simulink model "ReachTask_Perturb"  (R2022b)
settings: Solver=FixedStepDiscrete  StartTime=0.0  StopTime=Inf  FixedStep=0.001  RelTol=1e-3  EnableMultiTasking=on
PreLoadFcn:
  | parambus = Simulink.Bus;
  | idx = 0;
  | 
  | idx = idx + 1;
  | parambus.Elements(idx) = Simulink.BusElement;
  | parambus.Elements(idx).Name = 'ScreenOn';
  | parambus.Elements(idx).DataType = 'uint8';
  | parambus.Elements(idx).Dimensions = [1, 1];
  | 
  | idx = idx + 1;
  | parambus.Elements(idx) = Simulink.BusElement;
  | parambus.Elements(idx).Name = 'DelayPeriod';
  | parambus.Elements(idx).DataType = 'uint16';
  | parambus.Elements(idx).Dimensions = [1, 2];
  | 
  | idx = idx + 1;
  | parambus.Elements(idx) = Simulink.BusElement;
  | parambus.Elements(idx).Name = 'TargetHoldTime';
  | parambus.Elements(idx).DataType = 'uint16';
  | parambus.Elements(idx).Dimensions = [1, 1];
  | 
  | idx = idx + 1;
  | parambus.Elements(idx) = Simulink.BusElement;
  | parambus.Elements(idx).Name = 'TargetScaling';
  | parambus.Elements(idx).DataType = 'uint8';
  | parambus.Elements(idx).Dimensions = [1, 1];
  | 
  | idx = idx + 1;
  | parambus.Elements(idx) = Simulink.BusElement;
  | parambus.Elements(idx).Name = 'TrialTimeout';
  | parambus.Elements(idx).DataType = 'uint16';
  | parambus.Elements(idx).Dimensions = [1, 1];
  | 
  | 
  | FileLoggerEntry = Simulink.Bus;
  | FileLoggerEntry.Elements(1) = Simulink.BusElement;
  | FileLoggerEntry.Elements(1).Name = 'FileType';
  | FileLoggerEntry.Elements(1).DataType = 'uint8';
  | FileLoggerEntry.Elements(1).Dimensions = [1, 1];
  | FileLoggerEntry.Elements(2) = Simulink.BusElement;
  | FileLoggerEntry.Elements(2).Name = 'FieldName';
  | FileLoggerEntry.Elements(2).DataType = 'uint8';
  | FileLoggerEntry.Elements(2).Dimensions = [1, 20];
  | FileLoggerEntry.Elements(3) = Simulink.BusElement;
  | FileLoggerEntry.Elements(3).Name = 'DataType';
  | FileLoggerEntry.Elements(3).DataType = 'uint8';
  | FileLoggerEntry.Elements(3).Dimensions = [1, 6];
  | FileLoggerEntry.Elements(4) = Simulink.BusElement;
  | FileLoggerEntry.Elements(4).Name = 'NumElements';
  | FileLoggerEntry.Elements(4).DataType = 'uint8';
  | FileLoggerEntry.Elements(4).Dimensions = [1, 1];
  | FileLoggerEntry.Elements(5) = Simulink.BusElement;
  | FileLoggerEntry.Elements(5).Name = 'Data';
  | FileLoggerEntry.Elements(5).DataType = 'double';
  | FileLoggerEntry.Elements(5).Dimensions = [1, 255];
undefined symbols (not defined in the file): IO397
libraries: slrealtimeiplib x7, speedgoatlib_fpga_spi x1, speedgoatlib_fpga x1
settings Model: Creator=irwin  LastModifiedBy=irwin
settings SolverCC: ConcurrentTasks=on  AlgebraicLoopSolver=TrustRegion  PositivePriorityOrder=on  InsertRTBMode=Never (minimum delay)
settings DataIOCC: SaveFormat=Array  SaveState=on  SignalLoggingName=logsOut
settings OptimizationCC: BlockReduction=off  BooleanDataType=off  OptimizeBlockIOStorage=off  BufferReuse=off  GlobalBufferReuse=off  ExpressionFolding=off  LocalBlockOutputs=off  InitFltsAndDblsToZero=on  OptimizeDataStoreBuffers=off  BusAssignmentInplaceUpdate=off
settings DebuggingCC: SaveWithParameterizedLinksMsg=none  UnderspecifiedInitializationDetection=Classic  MergeDetectMultiDrivingBlocksExec=none  CheckExecutionContextPreStartOutputMsg=on  SignalResolutionControl=TryResolveAllWithWarning  TasksWithSamePriorityMsg=none  UnconnectedInputMsg=warning  UnconnectedOutputMsg=warning  UnconnectedLineMsg=warning  SFUnexpectedBacktrackingDiag=warning  SFNoUnconditionalDefaultTransitionDiag=warning  SFExecutionAtInitializationDiag=none  SFMachineParentedDataDiag=warning  ArithmeticOperatorsInVariantConditions=warning
settings HardwareCC: ProdBitPerLong=64  ProdLongLongMode=on  ProdHWDeviceType=Intel->x86-64 (Linux 64)
settings ModelReferenceCC: EnableRefExpFcnMdlSchedulingChecks=on  PropagateSignalLabelsOutOfModel=off
settings SFSimCC: SimUseLocalCustomCode=off  SimTargetLang=C++
settings RTWCC: Description=Simulink Real-Time  SystemTargetFile=slrealtime.tlc  TemplateMakefile=slrealtime_default_tmf  RTWUseLocalCustomCode=off  Toolchain=Simulink Real-Time Toolchain  BuildConfiguration=Faster Runs  CodeExecutionProfiling=on  TargetLang=C++  DLArmComputeVersion=19.05
settings CodeAppCC: StateflowObjectComments=on
settings SimulinkRealTimeTargetCC: MATLABClassNameForMDSCustomization=Simulink.SoftwareTarget.GRTCustomization  UseGCCFastMath=on
settings ConfigComp: CovMetricSettings=dw  CovSaveCumulativeToWorkspaceVar=on  CovSaveSingleToWorkspaceVar=on  CovExternalEMLEnable=off  CovSFcnEnable=off

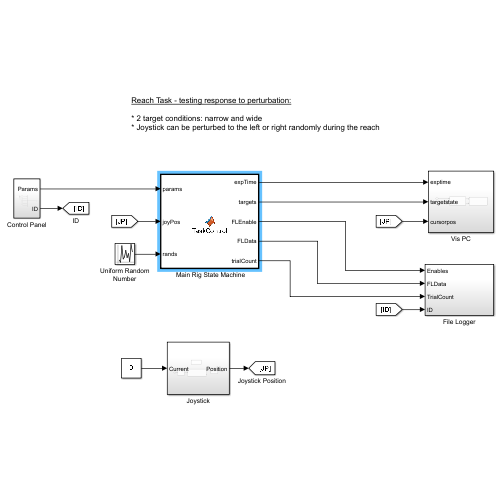
[thumbnail: Simulink's stored preview of the top-level diagram]
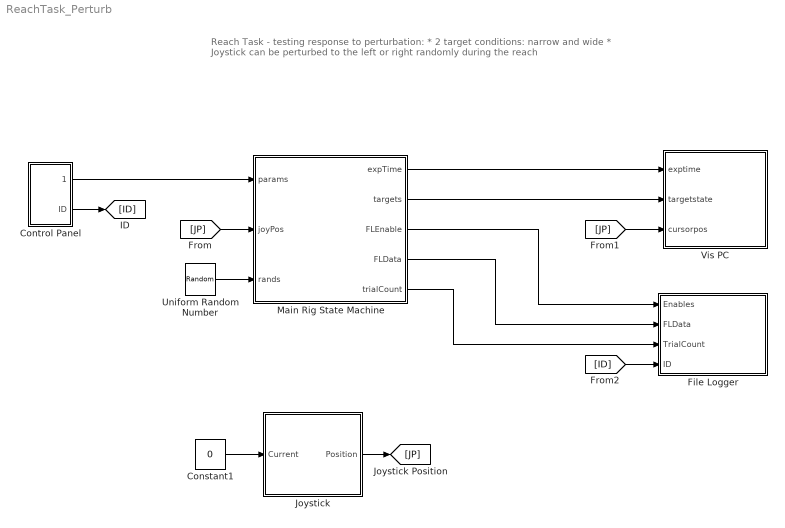
== system ReachTask_Perturb ==
  note: Reach Task - testing response to perturbation:
      |
      | * 2 target conditions: narrow and wide
      | * Joystick can be perturbed to the left or right randomly during the reach
  " Main Rig State Machine" : MATLAB Function  TreatAsAtomicUnit=on
  Constant1 : Constant  Value=0  OutMin=-5  OutMax=5  OutDataTypeStr=single
  Control Panel : Subsystem
  File Logger : Subsystem
  Joystick : Subsystem
  Uniform Random Number : UniformRandomNumber  Minimum=[0, 0, 0]  Maximum=[2, 2, 1]  SampleTime=.001
  Vis PC : Subsystem
  wires:
  " Main Rig State Machine"/1(expTime) -> Vis PC/1(exptime)
  " Main Rig State Machine"/2(targets) -> Vis PC/2(targetstate)
  " Main Rig State Machine"/3(FLEnable) -> File Logger/1(Enables)
  " Main Rig State Machine"/4(FLData) -> File Logger/2(FLData)
  " Main Rig State Machine"/5(trialCount) -> File Logger/3(TrialCount)
  [JP] -> " Main Rig State Machine"/2(joyPos)
  [JP] -> Vis PC/3(cursorpos)
  Control Panel/2(ID) -> [ID]
  [ID] -> File Logger/4(ID)
  Control Panel/1(Params) -> " Main Rig State Machine"/1(params)
  Uniform Random Number/1 -> " Main Rig State Machine"/3(rands)
  Joystick/1(Position) -> [JP]
  Constant1/1 -> Joystick/1(Current)

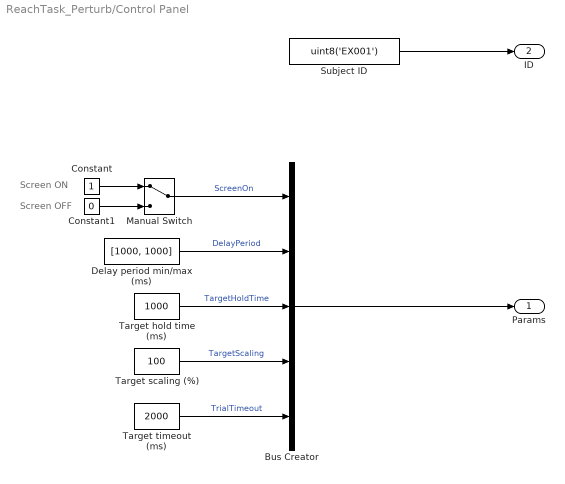
== system ReachTask_Perturb/Control Panel ==
  note: Screen ON
  note: Screen OFF
  Bus Creator : BusCreator  Inputs=5  OutDataTypeStr=Bus: parambus  NonVirtualBus=on
      settings: InheritFromInputs=off
  Constant : Constant  OutDataTypeStr=uint8
  Constant1 : Constant  Value=0  OutDataTypeStr=uint8
  Delay period min/max (ms) : Constant  Value=[1000, 1000]  OutDataTypeStr=uint16
  Manual Switch : ManualSwitch
  Subject ID : Constant  Value=uint8('EX001')  OutDataTypeStr=uint8
  Target hold time (ms) : Constant  Value=1000  OutDataTypeStr=uint16
  Target scaling (%) : Constant  Value=100  OutDataTypeStr=uint8
  Target timeout (ms) : Constant  Value=2000  OutDataTypeStr=uint16
  Params : Outport
  ID : Outport  Port=2
  wires:
  Delay period min/max (ms)/1 -> Bus Creator/2  "DelayPeriod"
  Manual Switch/1 -> Bus Creator/1  "ScreenOn"
  Constant1/1 -> Manual Switch/2
  Constant/1 -> Manual Switch/1
  Bus Creator/1 -> Params/1
  Target hold time (ms)/1 -> Bus Creator/3  "TargetHoldTime"
  Subject ID/1 -> ID/1
  Target timeout (ms)/1 -> Bus Creator/5  "TrialTimeout"
  Target scaling (%)/1 -> Bus Creator/4  "TargetScaling"

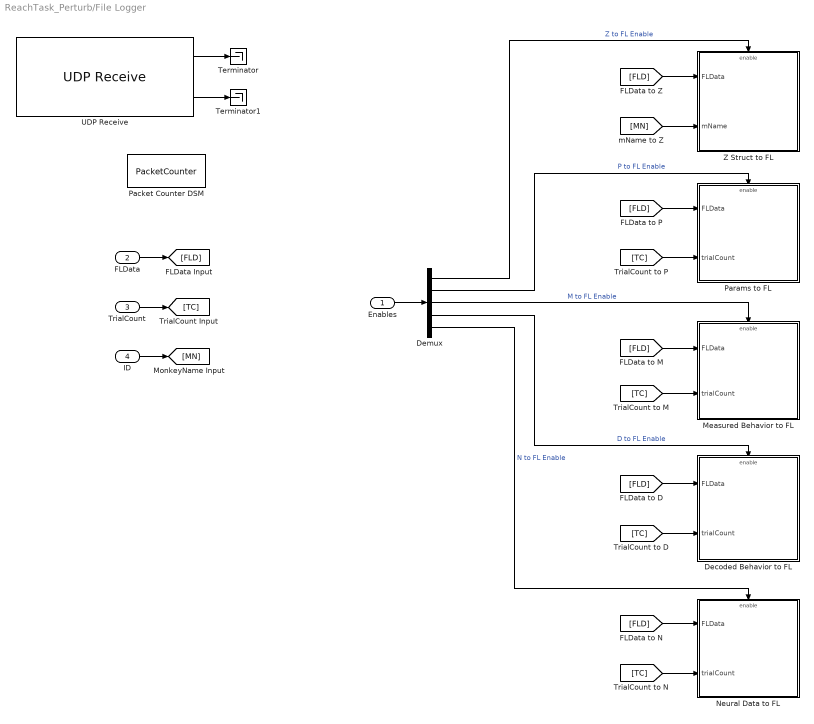
== system ReachTask_Perturb/File Logger ==
  Enables : Inport  OutDataTypeStr=uint8  PortDimensions=[1 5]
  FLData : Inport  Port=2  OutDataTypeStr=Bus: FileLoggerEntry
  TrialCount : Inport  Port=3
  ID : Inport  Port=4
  Decoded Behavior to FL : Subsystem
  Demux : Demux  Outputs=5
  Measured Behavior to FL : Subsystem
  Neural Data to FL : Subsystem
  Packet Counter DSM : DataStoreMemory  DataStoreName=PacketCounter  WriteAfterWriteMsg=warning  ShowAdditionalParam=off  OutDataTypeStr=uint32  Dimensions=1
  Params to FL : Subsystem
  Terminator : Terminator
  Terminator1 : Terminator
  UDP Receive : slrealtimeiplib/UDP Receive  useHostTargetConn=off  ipAddress='192.168.8.1'  localPort=11114  rcvWidth=16  rcvFmAny=off  fmAddress='192.168.8.7'  sampleTime=-1  enableMessage=off  maxPackets=1
  Z Struct to FL : Subsystem
  wires:
  TrialCount/1 -> [TC]
  FLData/1 -> [FLD]
  [FLD] -> Z Struct to FL/1(FLData)
  [FLD] -> Params to FL/1(FLData)
  [FLD] -> Measured Behavior to FL/1(FLData)
  [FLD] -> Decoded Behavior to FL/1(FLData)
  [FLD] -> Neural Data to FL/1(FLData)
  [TC] -> Params to FL/2(trialCount)
  [TC] -> Measured Behavior to FL/2(trialCount)
  [TC] -> Decoded Behavior to FL/2(trialCount)
  [TC] -> Neural Data to FL/2(trialCount)
  Enables/1 -> Demux/1
  Demux/3 -> Measured Behavior to FL/Enable  "M to FL Enable"
  Demux/4 -> Decoded Behavior to FL/Enable  "D to FL Enable"
  Demux/5 -> Neural Data to FL/Enable  "N to FL Enable"
  Demux/2 -> Params to FL/Enable  "P to FL Enable"
  Demux/1 -> Z Struct to FL/Enable  "Z to FL Enable"
  ID/1 -> [MN]
  [MN] -> Z Struct to FL/2(mName)
  UDP Receive/2 -> Terminator1/1
  UDP Receive/1 -> Terminator/1

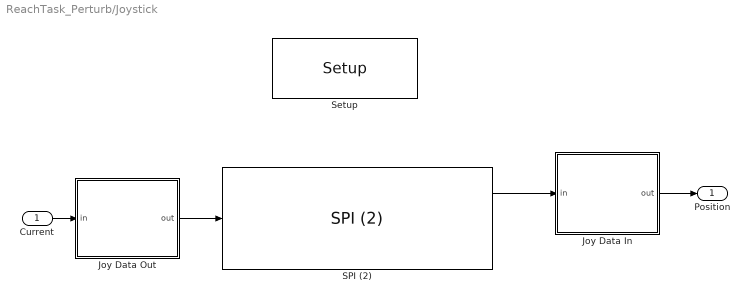
== system ReachTask_Perturb/Joystick ==
  Current : Inport
  Joy Data In : MATLAB Function  TreatAsAtomicUnit=on
  Joy Data Out : MATLAB Function  TreatAsAtomicUnit=on
  SPI (2) : speedgoatlib_fpga_spi/SPI (2)  id=1  chan=[1]  samp_time=.001  board=IO397-50k  pciSlot=-1  role=Master  sync_mode=off  multislave_mode=off  write_only=off  read_only=off  multislave_chan=[1]  cpol=[0]  cpha=[0]  frequency=[1e6]  frequency_eff=1e6  delay_start=[2e-6]  delay_start_eff=2e-6  delay_interword=[1e-6]  delay_interword_eff=1e-6  delay_stop=[1e-6]  delay_stop_eff=1e-6  delay_compensation=[100e-9]  delay_compensation_eff=106.7e-9  words_per_frame=[2]  dynamic_words_per_frame=off  bits_per_word=[16]  bit_shift_lsb_first=[0]  no_cs=off  clock_timeout=[1e-6]  clock_timeout_eff=1E-06
      settings: SourceProductName=Simulink Real-Time: Speedgoat I/O Blockset
  Setup : speedgoatlib_fpga/Setup/Setup  board=IO397-50k  id=1  device_id=1  frontIO=None  rearIO=None  bitstreamFile=speedgoat_IO397_50k_Comms.mat  rev=4.000000  timestamp_string=18/02/22 13:58:38  fpgaFreq=75 MHz  fpgaTick=13.33 ns  ProgSpiFlash=off  ProgBPIFlash=off  pciSlot=-1  PullRPort0=pull-up 3.3V  VioPort0=3.3V  PullRPort1=pull-up 3.3V  VioPort1=3.3V  PullRPort2=pull-up 3.3V  VioPort2=3.3V  PullRPort3=pull-up 3.3V  VioPort3=3.3V  PullRPort4=pull-up 3.3V  VioPort4=3.3V  PullRPort5=pull-up 3.3V  VioPort5=3.3V  PullRPort6=pull-up 3.3V  VioPort6=3.3V  diffLineTermination_rear1=on  diffLineTermination_rear2=on  diffLineTermination_rear3=on  diffLineTermination_rear4=on  diffLineTermination_rear5=on  diffLineTermination_rear6=on  diffLineTermination_rear7=on  diffLineTermination_rear8=on  PullRPort15=pull-up 3.3V  PullRPort31=pull-up 3.3V  PullRPort47=pull-up 3.3V  PullRPort63=pull-up 3.3V  diffLineTermination_1=on  diffLineTermination_2=on  diffLineTermination_3=on  diffLineTermination_4=on  diffLineTermination_5=on  diffLineTermination_6=on  diffLineTermination_7=on  diffLineTermination_8=on
      settings: SourceProductName=Simulink Real-Time: Speedgoat I/O Blockset
  Position : Outport
  wires:
  Joy Data Out/1(out) -> SPI (2)/1
  SPI (2)/1 -> Joy Data In/1(in)
  Current/1 -> Joy Data Out/1(in)
  Joy Data In/1(out) -> Position/1

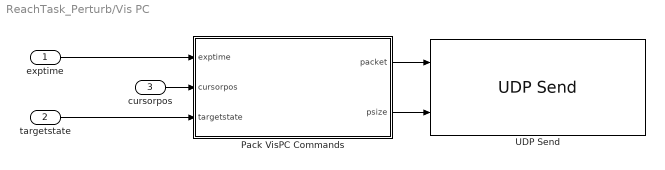
== system ReachTask_Perturb/Vis PC ==
  exptime : Inport
  targetstate : Inport  Port=2
  cursorpos : Inport  Port=3
  Pack VisPC Commands : MATLAB Function  TreatAsAtomicUnit=on
  UDP Send : slrealtimeiplib/UDP Send  useHostTargetConn=off  toAddress='192.168.11.6'  toPort=11114  sampleTime=-1  enableMessage=off  ipAddress='192.168.11.1'  localPort=11114
  wires:
  cursorpos/1 -> Pack VisPC Commands/2(cursorpos)
  Pack VisPC Commands/1(packet) -> UDP Send/1
  Pack VisPC Commands/2(psize) -> UDP Send/2
  targetstate/1 -> Pack VisPC Commands/3(targetstate)
  exptime/1 -> Pack VisPC Commands/1(exptime)

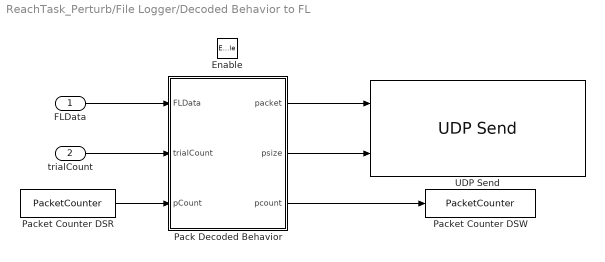
== system ReachTask_Perturb/File Logger/Decoded Behavior to FL ==
  FLData : Inport
  trialCount : Inport  Port=2
  Enable : EnablePort
  Pack Decoded Behavior : MATLAB Function  TreatAsAtomicUnit=on
  Packet Counter DSR : DataStoreRead  DataStoreName=PacketCounter  SampleTime=.001  IndexOptions=Index vector (dialog)  Indices=1  OutputSizes=1
  Packet Counter DSW : DataStoreWrite  DataStoreName=PacketCounter  IndexOptions=Index vector (dialog)  Indices=1  OutputSizes=1
  UDP Send : slrealtimeiplib/UDP Send  useHostTargetConn=off  toAddress='192.168.8.7'  toPort=11114  sampleTime=-1  enableMessage=off  ipAddress='192.168.8.1'  localPort=11114
  wires:
  FLData/1 -> Pack Decoded Behavior/1(FLData)
  trialCount/1 -> Pack Decoded Behavior/2(trialCount)
  Packet Counter DSR/1 -> Pack Decoded Behavior/3(pCount)
  Pack Decoded Behavior/1(packet) -> UDP Send/1
  Pack Decoded Behavior/3(pcount) -> Packet Counter DSW/1
  Pack Decoded Behavior/2(psize) -> UDP Send/2

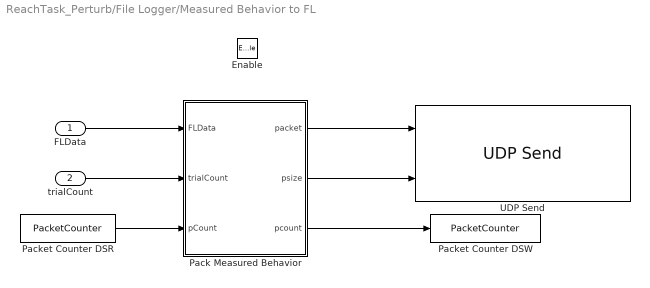
== system ReachTask_Perturb/File Logger/Measured Behavior to FL ==
  FLData : Inport
  trialCount : Inport  Port=2
  Enable : EnablePort
  Pack Measured Behavior : MATLAB Function  TreatAsAtomicUnit=on
  Packet Counter DSR : DataStoreRead  DataStoreName=PacketCounter  SampleTime=.001  IndexOptions=Index vector (dialog)  Indices=1  OutputSizes=1
  Packet Counter DSW : DataStoreWrite  DataStoreName=PacketCounter  IndexOptions=Index vector (dialog)  Indices=1  OutputSizes=1
  UDP Send : slrealtimeiplib/UDP Send  useHostTargetConn=off  toAddress='192.168.8.7'  toPort=11114  sampleTime=-1  enableMessage=off  ipAddress='192.168.8.1'  localPort=11114
  wires:
  FLData/1 -> Pack Measured Behavior/1(FLData)
  trialCount/1 -> Pack Measured Behavior/2(trialCount)
  Packet Counter DSR/1 -> Pack Measured Behavior/3(pCount)
  Pack Measured Behavior/3(pcount) -> Packet Counter DSW/1
  Pack Measured Behavior/1(packet) -> UDP Send/1
  Pack Measured Behavior/2(psize) -> UDP Send/2

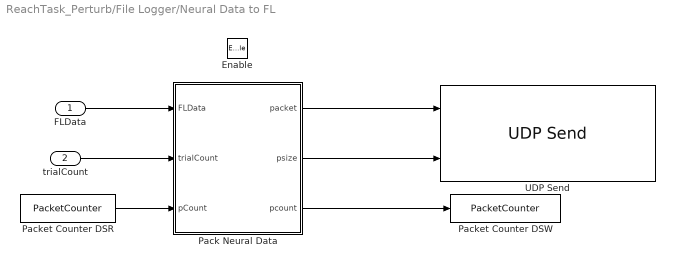
== system ReachTask_Perturb/File Logger/Neural Data to FL ==
  FLData : Inport
  trialCount : Inport  Port=2
  Enable : EnablePort
  Pack Neural Data : MATLAB Function  TreatAsAtomicUnit=on
  Packet Counter DSR : DataStoreRead  DataStoreName=PacketCounter  SampleTime=.001  IndexOptions=Index vector (dialog)  Indices=1  OutputSizes=1
  Packet Counter DSW : DataStoreWrite  DataStoreName=PacketCounter  IndexOptions=Index vector (dialog)  Indices=1  OutputSizes=1
  UDP Send : slrealtimeiplib/UDP Send  useHostTargetConn=off  toAddress='192.168.8.7'  toPort=11114  sampleTime=-1  enableMessage=off  ipAddress='192.168.8.1'  localPort=11114
  wires:
  FLData/1 -> Pack Neural Data/1(FLData)
  trialCount/1 -> Pack Neural Data/2(trialCount)
  Packet Counter DSR/1 -> Pack Neural Data/3(pCount)
  Pack Neural Data/3(pcount) -> Packet Counter DSW/1
  Pack Neural Data/1(packet) -> UDP Send/1
  Pack Neural Data/2(psize) -> UDP Send/2

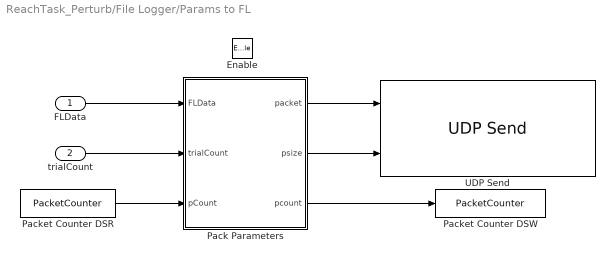
== system ReachTask_Perturb/File Logger/Params to FL ==
  FLData : Inport
  trialCount : Inport  Port=2
  Enable : EnablePort
  Pack Parameters : MATLAB Function  TreatAsAtomicUnit=on
  Packet Counter DSR : DataStoreRead  DataStoreName=PacketCounter  SampleTime=.001  IndexOptions=Index vector (dialog)  Indices=1  OutputSizes=1
  Packet Counter DSW : DataStoreWrite  DataStoreName=PacketCounter  IndexOptions=Index vector (dialog)  Indices=1  OutputSizes=1
  UDP Send : slrealtimeiplib/UDP Send  useHostTargetConn=off  toAddress='192.168.8.7'  toPort=11114  sampleTime=-1  enableMessage=off  ipAddress='192.168.8.1'  localPort=11114
  wires:
  FLData/1 -> Pack Parameters/1(FLData)
  trialCount/1 -> Pack Parameters/2(trialCount)
  Packet Counter DSR/1 -> Pack Parameters/3(pCount)
  Pack Parameters/1(packet) -> UDP Send/1
  Pack Parameters/2(psize) -> UDP Send/2
  Pack Parameters/3(pcount) -> Packet Counter DSW/1

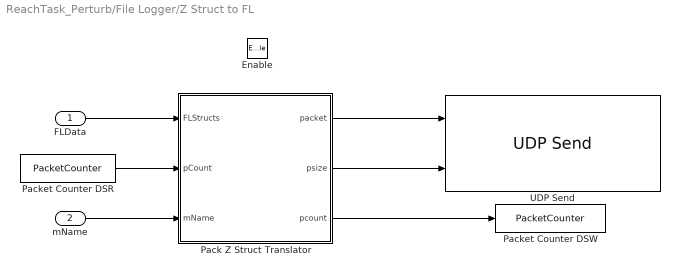
== system ReachTask_Perturb/File Logger/Z Struct to FL ==
  FLData : Inport
  mName : Inport  Port=2
  Enable : EnablePort
  Pack Z Struct Translator : MATLAB Function  TreatAsAtomicUnit=on
  Packet Counter DSR : DataStoreRead  DataStoreName=PacketCounter  SampleTime=.001  IndexOptions=Index vector (dialog)  Indices=1  OutputSizes=1
  Packet Counter DSW : DataStoreWrite  DataStoreName=PacketCounter  IndexOptions=Index vector (dialog)  Indices=1  OutputSizes=1
  UDP Send : slrealtimeiplib/UDP Send  useHostTargetConn=off  toAddress='192.168.8.7'  toPort=11114  sampleTime=-1  enableMessage=off  ipAddress='192.168.8.1'  localPort=11114
  wires:
  FLData/1 -> Pack Z Struct Translator/1(FLStructs)
  Packet Counter DSR/1 -> Pack Z Struct Translator/2(pCount)
  mName/1 -> Pack Z Struct Translator/3(mName)
  Pack Z Struct Translator/3(pcount) -> Packet Counter DSW/1
  Pack Z Struct Translator/1(packet) -> UDP Send/1
  Pack Z Struct Translator/2(psize) -> UDP Send/2

== matlab function ReachTask_Perturb/Vis PC/Pack VisPC Commands ==
  data: exptime input; cursorpos input; targetstate input; packet output; psize output
%
% targetstate [4 x 3]: state of each target (home, narrow, wide)
%   * Row 1: Target visibility
%   * Row 2: Target hit indicators
%   * Row 3: Target sizes
%   * Row 4: Target fill indicator
%
function [packet, psize] = CreateVisPacket(exptime, cursorpos, targetstate)

persistent position scale color visibility fill ...
           hitcolor basecolor ...
           hometarget reachtarget_narrow reachtarget_wide cursor

if (isempty(position))

    % definitions for available objects:
    hometarget = uint8(0);
    reachtarget_narrow = uint8(1);
    reachtarget_wide = uint8(2);
    cursor = uint8(3);
    
    % definitions for available object properties:
    position = uint8(1);
    visibility = uint8(2);
    color = uint8(3);
    scale = uint8(4);
    fill = uint8(5);

    % default property values:
    hitcolor = uint8([0, 0, 255]);
    basecolor = uint8([255, 0, 0]);

end

% Visibility:
pvisible = zeros(1,3*size(targetstate, 2), 'uint8');
for i = 1:size(targetstate,2)
    pvisible((i-1)*3 + 1) = i-1;
    pvisible((i-1)*3 + 2) = visibility;
    pvisible((i-1)*3 + 3) = targetstate(1,i);
end

% Scaling:
pscaling = zeros(1,3*size(targetstate, 2), 'uint8');
for i = 1:size(targetstate,2)
    pscaling((i-1)*3 + 1) = i-1;
    pscaling((i-1)*3 + 2) = scale;
    pscaling((i-1)*3 + 3) = targetstate(3,i);
end

% Color:
pcolor = zeros(1,5*size(targetstate, 2), 'uint8');
for i = 1:size(targetstate,2)
    pcolor((i-1)*5 + 1) = i-1;
    pcolor((i-1)*5 + 2) = color;
    if (targetstate(2,i))
        pcolor(((i-1)*5 + 3):i*5) = hitcolor;
    else
        pcolor(((i-1)*5 + 3):i*5) = basecolor;
    end
end

% Fill:
pfill = zeros(1,3*size(targetstate, 2), 'uint8');
for i = 1:size(targetstate,2)
    pfill((i-1)*3 + 1) = i-1;
    pfill((i-1)*3 + 2) = fill;
    pfill((i-1)*3 + 3) = targetstate(4,i);
end

% Position:
pposition = zeros(1,6,'uint8');
pposition(1) = cursor;
pposition(2) = position;
pposition(3:end) = typecast(cursorpos, 'uint8');

% Collect into single packet, compute size, then pad to final size:
temppacket = [typecast(exptime, 'uint8'), pvisible, pscaling, pcolor, pfill, pposition];
psize = length(temppacket);
packet = [temppacket, zeros(1,1500 - psize, 'uint8')];

== matlab function ReachTask_Perturb/ Main Rig State Machine ==
  data: expTime output uint32 size=1; params input; joyPos input; rands input; targets output; FLEnable output; FLData output Bus: FileLoggerEntry; trialCount output
function [expTime, targets, FLEnable, FLData, trialCount] = TaskControl(params, joyPos, rands)

persistent exp_state trial_state exp_time trial_time trial_count intparams extparams...
           targpos targrad prev_time FLStruct

if (isempty(exp_state))
    exp_state = uint8(0);           % Experiment state variable
    trial_state = uint8(0);         % Trial state variable
    exp_time = uint32(0);           % Current experiment time
    trial_time = uint32(0);         % Current trial time
    trial_count = uint16(0);        % Count of the trials in the current run
    extparams = params;             % Initialize parameters to incoming struct
    prev_time = double(-1);         % Marker for timing
    FLStruct = genFLStruct();       % Struct array for File Logger data

    intparams = struct('TrialType', uint8(0), ...           % 2 trial conditions - normal/perturbed
                       'TargetType', uint8(0), ...           % 2 targets - narrow/wide
                       'DelayTime', uint16(0), ...          % delay period (ms)
                       'TrialSuccess', uint8(0), ...        % trial success indicator
                       'BlankTrial', uint8(0), ...          % indicator that screen was turned off
                       'TargetHit', zeros(1,3,'uint8'), ... % hit indicators for each target + home
                       'TargetFill', ones(1,3,'uint8'), ... % fill indicators for each target + home
                       'TargetVis', ones(1,3,'uint8'));      % visbility indicators for each target + home
    
    targpos = [800, 800;
               400, 100;
               1200, 100];
    targrad = 50;

end

%%%%%%%%%%%%%%%%%%%%%%%%%%%%%%% Defines %%%%%%%%%%%%%%%%%%%%%%%%%%%%%%%%%%%

% Trial states:
tstate = struct('INIT',  uint8(0), ...
                'HOME',  uint8(1), ...
                'REACH', uint8(3), ...
                'HOLD',  uint8(4), ...
                'DONE',  uint8(5), ...
                'BLANK', uint8(6));

% Trial types:
trialtype = struct('NORMAL', uint8(0), ...
               'PERTURB', uint8(1));

% Target types:
targettype = struct('NARROW', uint8(0), ...
                    'WIDE', uint8(1));

% File Logger TX enables:
fenable = struct('ZENABLE', uint8(1), ...
                 'TENABLE', uint8(2), ...
                 'MENABLE', uint8(3), ...
                 'DENABLE', uint8(4), ...
                 'NENABLE', uint8(5));

%%%%%%%%%%%%%%%%%%%%%%%%% Per-timestep updates %%%%%%%%%%%%%%%%%%%%%%%%%%%%

exp_time = exp_time + uint32(1);     % Update simulation time (1 ms per function call)
trial_time = trial_time + 1; % Update trial time

FLEnable = zeros(1,5,'uint8'); % Initialize file logger enables for this timestep

% Test for hit targets:
intparams.TargetHit = uint8([0,0,0]);
for i = 1:3
    if (~intparams.TargetVis(i))
        continue;
    end
    if (sqrt(sum((single(joyPos) - targpos(i,:)).^2)) <= targrad*double(extparams.TargetScaling)/100)
        intparams.TargetHit(i) = uint8(1);
    else
        intparams.TargetHit(i) = uint8(0);
    end
end

%%%%%%%%%%%%%%%%%%%%%%% Stateflow switch statement %%%%%%%%%%%%%%%%%%%%%%%%

switch exp_state % Primary taskflow (experiment)
    case 0      % Initializing the File Logger
        
        %Send Z struct translator to File Logger:
        FLEnable(fenable.ZENABLE) = uint8(1);
        
        trial_state = tstate.INIT;
        exp_state = uint8(1);

    case 1      % Run the experiment
        switch trial_state % Secondary taskflow (per trial)

            case tstate.INIT

                %Pick up changes to trial parameters:
                extparams = params;
                
                % Determine the trial and target types:
                if (rands(1) < 1)
                    intparams.TrialType = trialtype.NORMAL;
                else
                    intparams.TrialType = trialtype.PERTURB;
                end
                if (rands(2) < 1)
                    intparams.TargetType = targettype.NARROW;
                else
                    intparams.TargetType = targettype.WIDE;
                end
                
                % Determine delay period time:
%                 intparams.DelayTime = uint16(rands(3)*double(diff(extparams.DelayPeriod)) + double(extparams.DelayPeriod(1)));

                % Reset target vis info:
                intparams.TargetHit = zeros(1,3,'uint8');
                intparams.TargetFill = ones(1,3,'uint8');
                intparams.TargetVis = uint8([1, 0, 0]); % show HOME target

                % Blank recording trial according to screen selection in Control Panel:
                intparams.BlankTrial = uint8(~extparams.ScreenOn);
                
                % Update File Logger struct with new trial params:
                FLStruct = updateFLParams(FLStruct, extparams, intparams);
                
                % Send trial parameters to File Logger:
                FLEnable(fenable.TENABLE) = uint8(1);
                
                if (intparams.BlankTrial)
                    trial_state = tstate.BLANK;
                else
                    trial_state = tstate.HOME;
                end

                trial_count = trial_count + uint16(1);
                trial_time = uint32(0);

            case tstate.HOME

                % If cursor in home target, test for complete hold:
                if (intparams.TargetHit(1))
                    if (prev_time < 0)
                        prev_time = double(exp_time);
                    end
                    if (exp_time - prev_time >= extparams.TargetHoldTime)
                        trial_state = tstate.REACH;
                        if (intparams.TargetType == targettypes.NARROW)
                            intparams.TargetVis = uint8([0, 1, 0]); % show NARROW target
                        else
                            intparams.TargetVis = uint8([0, 0, 1]); % show WIDE target
                        end

                    end
                else
                    prev_time = double(-1);
                end
                
                % Skip to a blank trial state if requested:
                if (~extparams.ScreenOn)
                    intparams.BlankTrial = uint8(1);
                    trial_state = tstate.BLANK;
                end

                %Update behavior/neural File Logger structs:
                FLStruct = updateFLData(FLStruct, joyPos, [], [], exp_time);
                
                %Send measured behavior + Neural to File Logger:
                FLEnable([fenable.MENABLE,fenable.NENABLE]) = uint8(1);

            case tstate.DELAY

                % Determine which target(s) are visible:
%                 intparams.TargetFill(2:3) = uint8(0);
%                 if (intparams.TrialType == ttype.IMPLICIT)
%                     intparams.TargetVis(2:3) = uint8(1);
%                 else
%                     intparams.TargetVis(2+intparams.TargetType) = uint8(1);
%                 end
% 
%                 % Test for cursor in home target and complete delay period:
%                 if (intparams.TargetHit(1))
%                     if (exp_time - prev_time >= extparams.TargetHoldTime + intparams.DelayTime)
%                         intparams.TargetVis(1) = uint8(0);
%                         prev_time = double(-1);
%                         trial_state = tstate.REACH;
%                     end
%                 else
%                     prev_time = double(-1);
%                     trial_state = tstate.DONE;
%                     intparams.TrialSuccess = uint8(0);
%                 end

                % Skip to a blank trial state if requested:
                if (~extparams.ScreenOn)
                    intparams.BlankTrial = uint8(1);
                    trial_state = tstate.BLANK;
                end

                %Update behavior/neural File Logger structs:
                FLStruct = updateFLData(FLStruct, joyPos, [], [], exp_time);
                
                %Send measured behavior + Neural to File Logger:
                FLEnable([fenable.MENABLE,fenable.NENABLE]) = uint8(1);
            
            case tstate.REACH

                intparams.TargetFill(2:3) = uint8(1);
                
%                 if (intparams.TrialType == ttype.IMPLICIT)
%                     hit = intparams.TargetHit(2) | intparams.TargetHit(3);
%                 else
%                     hit = logical(intparams.TargetHit(2+intparams.TargetType));
%                 end
                
                if (any(intparams.TargetHit))
                    if (prev_time < 0)
                        prev_time = double(exp_time);
                    end
                    if (exp_time - prev_time >= extparams.TargetHoldTime)
                        prev_time = double(-1);
                        trial_state = tstate.DONE;
                        intparams.TrialSuccess = uint8(1);
                    end
                else
                    prev_time = double(-1);
                end

                if (trial_time >= extparams.TrialTimeout)
                    trial_state = tstate.DONE;
                    intparams.TrialSuccess = uint8(0);
                end

                % Skip to a blank trial state if requested:
                if (~extparams.ScreenOn)
                    intparams.BlankTrial = uint8(1);
                    trial_state = tstate.BLANK;
                end

                %Update behavior/neural File Logger structs:
                FLStruct = updateFLData(FLStruct, joyPos, [], [], exp_time);
                
                %Send measured behavior + Neural to File Logger:
                FLEnable([fenable.MENABLE,fenable.NENABLE]) = uint8(1);

            case tstate.DONE

                intparams.TargetHit = zeros(1,3,'uint8');
                intparams.TargetFill = ones(1,3,'uint8');
                intparams.TargetVis = zeros(1,3,'uint8');

                trial_state = tstate.INIT;

                % Send trial parameters to File Logger:
                FLEnable(fenable.TENABLE) = uint8(1);

            case tstate.BLANK

                intparams.TargetHit = zeros(1,3,'uint8');
                intparams.TargetFill = ones(1,3,'uint8');
                intparams.TargetVis = zeros(1,3,'uint8');

                if (trial_time >= extparams.TrialTimeout || extparams.ScreenOn)
                    trial_state = tstate.DONE;
                    intparams.TrialSuccess = uint8(0);
                end

                %Update behavior/neural File Logger structs:
                FLStruct = updateFLData(FLStruct, joyPos, [], [], exp_time);
                
                %Send measured behavior + Neural to File Logger:
                FLEnable([fenable.MENABLE,fenable.NENABLE]) = uint8(1);
        end
end


%%%%%%%%%%%%%%%%%%%%%%%% Assign Output Variables: %%%%%%%%%%%%%%%%%%%%%%%%%

expTime = exp_time;

FLData = FLStruct;

targets = [intparams.TargetVis; intparams.TargetHit; repelem(extparams.TargetScaling,1,3); intparams.TargetFill];

trialCount = trial_count;

end

%%%%%%%%%%%%%%%%%%%%%%%%%%% Helper Functions: %%%%%%%%%%%%%%%%%%%%%%%%%%%%%

% Initializes an array of structures for output to the File Logger:
function flStructs = genFLStruct()

%Set up initial structure for a FileLoggerEntry struct:
tempStructs = struct('FileType', uint8(0), 'FieldName', uint8(zeros(1,20)), ...
    'DataType', uint8(zeros(1,6)), 'NumElements', uint8(0), 'Data', zeros(1,255));

%Replicate N times (#params + #behavior [meas/dec] + #neural):
flStructs = repmat(tempStructs, 1, 10);

%File types:
ftype = struct('BEHAVIOR_MEAS', uint8(2), ...
               'BEHAVIOR_DEC', uint8(3), ...
               'DATA_NEUR', uint8(4), ...
               'PARAM_START', uint8(5), ...
               'PARAM_END', uint8(6));

%Set fieldnames, file types, data types:
flStructs(1) = getStruct(ftype.PARAM_START, 'DelayTime', 'uint16', 1, []);
flStructs(2) = getStruct(ftype.PARAM_START, 'TargetHoldTime', 'uint16', 1, []);
flStructs(3) = getStruct(ftype.PARAM_START, 'TargetScaling', 'uint8', 1, []);
flStructs(4) = getStruct(ftype.PARAM_START, 'TrialTimeout', 'uint16', 1, []);
flStructs(5) = getStruct(ftype.PARAM_START, 'TrialType', 'uint8', 1, []);
flStructs(6) = getStruct(ftype.PARAM_START, 'TargetType', 'uint8', 1, []);
flStructs(7) = getStruct(ftype.PARAM_END, 'BlankTrial', 'uint8', 1, []);
flStructs(8) = getStruct(ftype.PARAM_END, 'TrialSuccess', 'uint8', 1, []);
flStructs(9) = getStruct(ftype.BEHAVIOR_MEAS, 'JoyPosition', 'single', 2, []);
flStructs(10) = getStruct(ftype.BEHAVIOR_MEAS, 'ExperimentTime', 'single', 1, []);

end


% Updates the File Logger array with new parameters:
function flStructs = updateFLParams(flStruct_old, extparams, intparams)

%extparams = External, tunable parameters; intparams = Internal parameters.
%e.g. extparam1 = User-set TargetScaling, intparam1 = program-set TargetType.

flStructs = flStruct_old;
flStructs(1).Data(1:length(intparams.DelayTime))      = double(intparams.DelayTime);
flStructs(2).Data(1:length(extparams.TargetHoldTime)) = double(extparams.TargetHoldTime);
flStructs(3).Data(1:length(extparams.TargetScaling))  = double(extparams.TargetScaling);
flStructs(4).Data(1:length(extparams.TrialTimeout))   = double(extparams.TrialTimeout);
flStructs(5).Data(1:length(intparams.TrialType))      = double(intparams.TrialType);
flStructs(6).Data(1:length(intparams.TargetType))      = double(intparams.TargetType);
flStructs(7).Data(1:length(intparams.BlankTrial))     = double(intparams.BlankTrial);
flStructs(8).Data(1:length(intparams.TrialSuccess))   = double(intparams.TrialSuccess);

end

% Updates the File Logger array with new behavior/neural data:
function flStructs = updateFLData(flStruct_old, mBehavior, dBehavior, neural, eTime)

flStructs = flStruct_old;
flStructs(9).Data(1:length(mBehavior))  = double(mBehavior);
flStructs(10).Data(1:length(eTime))     = double(eTime);
end

% Helper function to create an FL struct from inputs:
function ret = getStruct(filetype,fieldname,datatype,numel,data)

ft = uint8(filetype);                                   % FileType
fn = uint8([fieldname, zeros(1,20-length(fieldname))]); % FieldName
dt = uint8([datatype, zeros(1,6-length(datatype))]);    % DataType
ne = uint8(numel);                                      % NumElements
d = double([data, zeros(1,255-length(data))]);          % Data

%Create and return structure:
ret = struct('FileType', ft, 'FieldName', fn, 'DataType', dt, 'NumElements', ne, 'Data', d);

end

== matlab function ReachTask_Perturb/Joystick/Joy Data Out ==
  data: in input single size=1; out output uint32 size=[1,2]
function out = FormatJoyDataOut(in)

out = uint32(typecast(single(in), 'uint16'));

== matlab function ReachTask_Perturb/Joystick/Joy Data In ==
  data: in input uint32 size=[1,2]; out output uint16 size=[1,2]
function out = FormatJoyDataIn(in)

in = single(in);

x = single((in(1) - 7650)/(12030 - 7650));
y = single((in(2) - 1950)/(5200 - 1950));

if (x < 0)
    x = single(0);
elseif (x > 1)
    x = single(1);
end

if (y < 0)
    y = single(0);
elseif (y > 1)
    y = single(1);
end

out = uint16([x,y].*[1600, 900]);

%  out = uint16(([x, y]/5).*[1600,900]);

== matlab function ReachTask_Perturb/File Logger/Z Struct to FL/Pack Z Struct Translator ==
  data: packet output uint8 size=[1,1500]; FLStructs input Bus: FileLoggerEntry; pCount input uint32 size=1; psize output double size=1; mName input uint8; pcount output uint32 size=1
% This translates the FileLoggerEntry struct array to a Z struct description
% string for the Z Struct Translator script to use at a later date.
%
% FL Packet:[packetCount(4b), packetType(1b), data(xb)]
%   -> First 2 bytes of non-ZPacket data are the trialCount
%
% Z Struct descriptor: 'fieldname1-datatype1-numElements1-fieldname2-...'
%
%   Written by Zach Irwin for the Chestek Lab, 2012
%%%%%%%%%%%%%%%%%%%%%%%%%%%%%%%%%%%%%%%%%%%%%%%%%%%%%%%%%%%%%%%%%%%%%%%%%%%

function [packet, psize, pcount] = genZPacket(FLStructs, pCount, mName)
%#codegen

sb = uint8('-'); % Spacer byte
headers = uint8([':P:'; ':M:'; ':D:'; ':N:']); % File Type headers

%Current packet size (with headers/monkey name, max size = 1500 bytes):
psize = double(4 + 1 + length(mName) + 1);

%Initialize packet (packetCount, packetType, mNameSize, mName, padding):
packet = uint8([typecast(uint32(pCount), 'uint8'), uint8(0), uint8(length(mName)), mName',zeros(1,1500-psize)]);

%Sort FLStructs into FileTypes (Params, mBehavior, dBehavior, Neural):
idxs = zeros(5,length(FLStructs));

for i = 1:length(FLStructs)

     switch FLStructs(i).FileType
         case 2 % Measured Behavior File Type
             idxs(2, nnz(idxs(2,:)) + 1) = i;
         case 3 % Decoded Behavior File Type
             idxs(3, nnz(idxs(3,:)) + 1) = i;
         case 4 % Neural Data File Type
             idxs(4, nnz(idxs(4,:)) + 1) = i;
         case 5 % Trial Begin Parameter File Type
             idxs(1, nnz(idxs(1,:)) + 1) = i;
         case 6 % Trial End Parameter File Type
             idxs(5, nnz(idxs(1,:)) + 1) = i;
     end
    
end

%Iterate through each File Type, add data to packet:
for i = 1:4
    
    % Collect structs for the current File Type:
    nidxs = idxs(i, :); % Current set of indices for ith File Type
    
    if (i == 1)
        nidxs5 = idxs(5,:); % Indices for the End Parameters File Type
        data = [FLStructs(nidxs(nidxs~=0)), FLStructs(nidxs5(nidxs5~=0))];
    else
        data = FLStructs(nidxs(nidxs ~= 0)); % Current File Type Structs
    end
    
    % Add correct File Type header:
    start = psize + uint16(1); stop = psize + uint16(3);
    packet(start:stop) = headers(i,:);
    
    % Update number of elements in the packet:
    psize = psize + double(3);
    
    % Iterate through the File Type structs & add to packet:
    for j = 1:length(data)
        
        % Recover non-NULL fieldName string:
        fname = data(j).FieldName(data(j).FieldName ~= 0);
        
        % Recover non-NULL dataType string:
        dtype = data(j).DataType(data(j).DataType ~= 0);
        
        % If either of these is empty, generate an error:
        if (isempty(fname) || isempty(dtype))
            error('An FLStruct FieldName or DataType is NULL. Don''t include extraneous FLStructs.');
        end
        
        % Recover numElements byte:
        numel = data(j).NumElements;
        
        % Size of all of these elements + 3 spacer bytes:
        inum = length(fname) + length(dtype) + length(numel) + 3;
        
        % Pack this set of bytes into the packet:
        start = psize + uint16(1); stop = psize + uint16(inum);
        packet(start:stop) = uint8([fname, sb, dtype, sb, numel, sb]);
        
        % Update number of elements in the packet:
        psize = psize + double(inum);
        
    end
    
end

% Update packet count:
pcount = pCount + uint32(1);

end

== matlab function ReachTask_Perturb/File Logger/Params to FL/Pack Parameters ==
  data: FLData input Bus: FileLoggerEntry; packet output uint8 size=[1,1500]; trialCount input uint16 size=1; pCount input uint32 size=1; psize output size=1; pcount output uint32 size=1
% This packs a vector of the trial parameters to send to the File Logger
%
% FL Packet:[runTime(4b), packetType(1b), data(xb)]
%   -> First 2 bytes of non-ZPacket data are the trialCount
%
%   Written by Zach Irwin for the Chestek Lab, 2012
%%%%%%%%%%%%%%%%%%%%%%%%%%%%%%%%%%%%%%%%%%%%%%%%%%%%%%%%%%%%%%%%%%%%%%%%%%%

function [packet, psize, pcount] = genPPacket(FLData, trialCount, pCount)
%#codegen

persistent prev_count

%This function gets called twice per trial, prev_count lets us know which
%type of trial parameters to send (FileType 5 or FileType 6)
if (isempty(prev_count))
    prev_count = -1;        
end

%Figure out which FileType to send:
if (prev_count == trialCount)
    ftype = 6;  %Send the Trial Wrap-up parameters
else
    ftype = 5;  %Send Trial Begin parameters
    prev_count = double(trialCount); %Reset count
end

%Convert runTime & trialCount to uint8 vectors:
rt = typecast(uint32(pCount), 'uint8');
tc = typecast(uint16(trialCount), 'uint8');

%Initialize packet vector [runTime(x4), packetType(x1), trialCount(x2), data(x1493)]:
packet = uint8([rt, uint8(ftype), tc, zeros(1,1493)]);

%Keep track of no. of bytes in the packet:
psize = double(7); %4 runTime bytes, 1 packetType byte, and 2 trialCount bytes

for i = 1:length(FLData)
    
    %Skip FLData structs without parameter data (fileType = 5 or 6):
   if (FLData(i).FileType ~= ftype)
       continue;
   end
   
   %Get non-zero data from struct:
   ddata = FLData(i).Data(1:FLData(i).NumElements); %Elements as doubles
   
   %Cast data to correct type, then uint8s for packing:
   type = char(FLData(i).DataType(FLData(i).DataType ~= 0));
   if (strcmp(type, 'uint8'))
       data = uint8(ddata);
   elseif (strcmp(type, 'int8'))
       data = typecast(int8(ddata),'uint8');
   elseif (strcmp(type, 'uint16'))
       data = typecast(uint16(ddata),'uint8');
   elseif (strcmp(type, 'int16'))
       data = typecast(int16(ddata),'uint8');
   elseif (strcmp(type, 'uint32'))
       data = typecast(uint32(ddata),'uint8');
   elseif (strcmp(type, 'int32'))
       data = typecast(int32(ddata),'uint8');
   elseif (strcmp(type, 'single'))
       data = typecast(single(ddata),'uint8');
   elseif (strcmp(type, 'double'))
       data = typecast(ddata,'uint8');
   else
       data = uint8(0); % Should never happen
   end
   
   %Add data to packet:
   start = psize + uint16(1); stop = psize + uint16(length(data));
   packet(start:stop) = data;
   
   %Update number of elements in the packet:
   psize = psize + double(length(data));
   
   if (psize > 1500)
       error('Packet size reached: P Packet type');
   end
   
end

%Update packet count:
pcount = pCount + uint32(1);
end

== matlab function ReachTask_Perturb/File Logger/Measured Behavior to FL/Pack Measured Behavior ==
  data: FLData input Bus: FileLoggerEntry; packet output uint8 size=[1,1500]; trialCount input uint16 size=1; pCount input uint32 size=1; psize output size=1; pcount output uint32 size=1
% This packs a vector of the measured behavior to send to the File Logger
%
% FL Packet:[runTime(4b), packetType(1b), data(xb)]
%   -> First 2 bytes of non-ZPacket data are the trialCount
%
%   Written by Zach Irwin for the Chestek Lab, 2012
%%%%%%%%%%%%%%%%%%%%%%%%%%%%%%%%%%%%%%%%%%%%%%%%%%%%%%%%%%%%%%%%%%%%%%%%%%%

function [packet, psize, pcount] = genMPacket(FLData, trialCount, pCount)
%#codegen

%Convert runTime & trialCount to uint8 vectors:
rt = typecast(uint32(pCount), 'uint8');
tc = typecast(uint16(trialCount), 'uint8');

%Initialize packet vector [runTime(x4), packetType(x1), trialCount(x2), data(x1493)]:
packet = uint8([rt, uint8(2), tc, zeros(1,1493)]);

%Keep track of no. of bytes in the packet:
psize = double(7); %4 runTime bytes, 1 packetType byte, and 2 trialCount bytes

for i = 1:length(FLData)
    
    %Skip FLData strucuts without meas. behavior data (fileType = 2):
   if (FLData(i).FileType ~= 2)
       continue;
   end
   
   %Get non-zero data from struct:
   ddata = FLData(i).Data(1:FLData(i).NumElements); %Elements as doubles
   
   %Cast data to correct type, then uint8s for packing:
   type = char(FLData(i).DataType(FLData(i).DataType ~= 0));
   if (strcmp(type, 'uint8'))
       data = uint8(ddata);
   elseif (strcmp(type, 'int8'))
       data = typecast(int8(ddata),'uint8');
   elseif (strcmp(type, 'uint16'))
       data = typecast(uint16(ddata),'uint8');
   elseif (strcmp(type, 'int16'))
       data = typecast(int16(ddata),'uint8');
   elseif (strcmp(type, 'uint32'))
       data = typecast(uint32(ddata),'uint8');
   elseif (strcmp(type, 'int32'))
       data = typecast(int32(ddata),'uint8');
   elseif (strcmp(type, 'single'))
       data = typecast(single(ddata),'uint8');
   elseif (strcmp(type, 'double'))
       data = typecast(ddata,'uint8');
   else
       data = uint8(0); % Should never happen
   end
   
   %Add data to packet:
   start = psize + uint16(1); stop = psize + uint16(length(data));
   packet(start:stop) = data;
   
   %Update number of elements in the packet:
   psize = psize + double(length(data));
   
   if (psize > 1500)
       error('Packet size reached: M Packet type');
   end
   
end

%Update packet count:
pcount = pCount + uint32(1);
end

== matlab function ReachTask_Perturb/File Logger/Decoded Behavior to FL/Pack Decoded Behavior ==
  data: FLData input Bus: FileLoggerEntry; packet output uint8 size=[1,1500]; trialCount input uint16 size=1; pCount input uint32 size=1; psize output size=1; pcount output uint32 size=1
% This packs a vector of the decoded behavior to send to the File Logger
%
% FL Packet:[runTime(4b), packetType(1b), data(xb)]
%   -> First 2 bytes of non-ZPacket data are the trialCount
%
%   Written by Zach Irwin for the Chestek Lab, 2012
%%%%%%%%%%%%%%%%%%%%%%%%%%%%%%%%%%%%%%%%%%%%%%%%%%%%%%%%%%%%%%%%%%%%%%%%%%%

function [packet, psize, pcount] = genDPacket(FLData, trialCount, pCount)
%#codegen

%Convert runTime & trialCount to uint8 vectors:
rt = typecast(uint32(pCount), 'uint8');
tc = typecast(uint16(trialCount), 'uint8');

%Initialize packet vector [runTime(x4), packetType(x1), trialCount(x2), data(x1493)]:
packet = uint8([rt, uint8(3), tc, zeros(1,1493)]);

%Keep track of no. of bytes in the packet:
psize = double(7); %4 runTime bytes, 1 packetType byte, and 2 trialCount bytes

for i = 1:length(FLData)
    
    %Skip FLData strucuts without dec. behavior data (fileType = 3):
   if (FLData(i).FileType ~= 3)
       continue;
   end
   
   %Get non-zero data from struct:
   ddata = FLData(i).Data(1:FLData(i).NumElements); %Elements as doubles
   
   %Cast data to correct type, then uint8s for packing:
   type = char(FLData(i).DataType(FLData(i).DataType ~= 0));
   if (strcmp(type, 'uint8'))
       data = uint8(ddata);
   elseif (strcmp(type, 'int8'))
       data = typecast(int8(ddata),'uint8');
   elseif (strcmp(type, 'uint16'))
       data = typecast(uint16(ddata),'uint8');
   elseif (strcmp(type, 'int16'))
       data = typecast(int16(ddata),'uint8');
   elseif (strcmp(type, 'uint32'))
       data = typecast(uint32(ddata),'uint8');
   elseif (strcmp(type, 'int32'))
       data = typecast(int32(ddata),'uint8');
   elseif (strcmp(type, 'single'))
       data = typecast(single(ddata),'uint8');
   elseif (strcmp(type, 'double'))
       data = typecast(ddata,'uint8');
   else
       data = uint8(0); % Should never happen
   end
   
   %Add data to packet:
   start = psize + uint16(1); stop = psize + uint16(length(data));
   packet(start:stop) = data;
   
   %Update number of elements in the packet:
   psize = psize + double(length(data));
   
   if (psize > 1500)
       error('Packet size reached: D Packet type');
   end
   
end

%Update packet count:
pcount = pCount + uint32(1);
end

== matlab function ReachTask_Perturb/File Logger/Neural Data to FL/Pack Neural Data ==
  data: FLData input Bus: FileLoggerEntry; packet output uint8 size=[1,1500]; trialCount input uint16 size=1; pCount input uint32 size=1; psize output size=1; pcount output uint32 size=1
    % This packs a vector of the Neural data to send to the File Logger
%
% FL Packet:[runTime(4b), packetType(1b), data(xb)]
%   -> First 2 bytes of non-ZPacket data are the trialCount
%
% *NOTE: Neural packets have an "end packet" character(255) as the last
% byte in the packet. This is to support variable length spike channels.
%
%   Written by Zach Irwin for the Chestek Lab, 2012
%%%%%%%%%%%%%%%%%%%%%%%%%%%%%%%%%%%%%%%%%%%%%%%%%%%%%%%%%%%%%%%%%%%%%%%%%%%

function [packet, psize, pcount] = genNPacket(FLData, trialCount, pCount)
%#codegen

%Convert runTime & trialCount to uint8 vectors:
rt = typecast(uint32(pCount), 'uint8');
tc = typecast(uint16(trialCount), 'uint8');

%Initialize packet vector [runTime(x4), packetType(x1), trialCount(x2), data(x1493)]:
packet = uint8([rt, uint8(4), tc, zeros(1,1493)]);

%Keep track of no. of bytes in the packet:
psize = double(7); %4 runTime bytes, 1 packetType byte, and 2 trialCount bytes

for i = 1:length(FLData)
    
    %Skip FLData structs without neural data (fileType = 4):
   if (FLData(i).FileType ~= 4)
       continue;
   end
   
   %Get non-zero data from struct:
   if (FLData(i).NumElements == 0)
        ddata = FLData(i).Data(FLData(i).Data ~= 0); %Elements as doubles
   else
        ddata = FLData(i).Data(1:FLData(i).NumElements); %Elements as doubles
   end
   
   %Cast data to correct type, then uint8s for packing:
   type = char(FLData(i).DataType(FLData(i).DataType ~= 0));
   if (strcmp(type, 'uint8'))
       data = uint8(ddata);
   elseif (strcmp(type, 'int8'))
       data = typecast(int8(ddata),'uint8');
   elseif (strcmp(type, 'uint16'))
       data = typecast(uint16(ddata),'uint8');
   elseif (strcmp(type, 'int16'))
       data = typecast(int16(ddata),'uint8');
   elseif (strcmp(type, 'uint32'))
       data = typecast(uint32(ddata),'uint8');
   elseif (strcmp(type, 'int32'))
       data = typecast(int32(ddata),'uint8');
   elseif (strcmp(type, 'single'))
       data = typecast(single(ddata),'uint8');
   elseif (strcmp(type, 'double'))
       data = typecast(ddata,'uint8');
   else
       data = uint8(0); % Should never happen
   end
   
   %Add data to packet:
   start = psize + uint16(1); stop = psize + uint16(length(data));
   packet(start:stop) = data;
   
   %Update number of elements in the packet:
   psize = psize + double(length(data));
   
   if (psize >= 1500)
       error('Packet size reached: N Packet type');
   end
   
end

%Add End Packet byte:
packet(psize+uint16(1)) = uint8(255);
psize = psize + double(1);

%Update packet count:
pcount = pCount + uint32(1);

end
